simulink model "simulate_FM_Passband_Model"  (R2021a)
settings: Solver=VariableStepAuto  StartTime=0.0  StopTime=0.1  RelTol=1e-3
InitFcn:
  | fs=4e3;
  | Ts=1/fs;
  | frameSize=1;
  | freqDev=250;
libraries: commanapbnd3 x2, dspsrcs4 x1
settings Model: Creator=Byung-Jun Jang  LastModifiedBy=user
settings SolverCC: AlgebraicLoopSolver=TrustRegion
settings DataIOCC: ReturnWorkspaceOutputs=off
settings DebuggingCC: SFMachineParentedDataDiag=warning  ArithmeticOperatorsInVariantConditions=warning
settings SFSimCC: SimUseLocalCustomCode=off  CustomCodeUndefinedFunction=UseInterfaceOnly
settings RTWCC: RTWUseLocalCustomCode=off
settings CodeAppCC: StateflowObjectComments=on
settings SimscapeCC: SimscapeNormalizeSystem=off

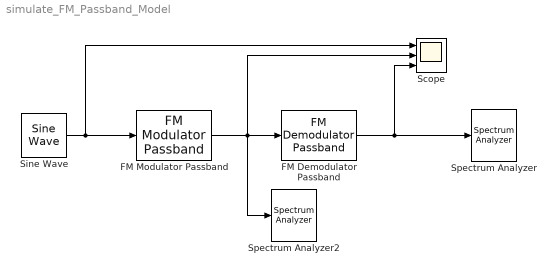
== system simulate_FM_Passband_Model ==
  FM Demodulator Passband : commanapbnd3/FM Demodulator Passband  Fc=2000  Ph=0  Kc=250  Ho=100
      settings: SourceProductBaseCode=CM
  FM Modulator Passband : commanapbnd3/FM Modulator Passband  Fc=2000  Ph=0  Kc=250
      settings: SourceProductBaseCode=CM
  Scope : Scope  NumInputPorts=3
  Sine Wave : dspsrcs4/Sine Wave  Amplitude=1  Frequency=300  Phase=0  SampleMode=Discrete  OutComplex=Real  CompMethod=Trigonometric fcn  TableSize=Speed  SampleTime=1/(fs*10)  SamplesPerFrame=frameSize  ResetState=Restart at time zero  OutputFrames=off  dataType=double  wordLen=16  udDataType=sfix(16)  fracBitsMode=Best precision  numFracBits=15  OutDataTypeStr=double  LastOutDataTypeStr=double
  Spectrum Analyzer : SpectrumAnalyzer
  Spectrum Analyzer2 : SpectrumAnalyzer
  wires:
  Sine Wave/1 -> FM Modulator Passband/1, Scope/1
  FM Demodulator Passband/1 -> Scope/3, Spectrum Analyzer/1
  FM Modulator Passband/1 -> Spectrum Analyzer2/1, Scope/2, FM Demodulator Passband/1
